simulink model "examples_of_product_block"  (R2021a)
settings: Solver=VariableStepAuto  StartTime=0.0  StopTime=1  RelTol=1e-3
settings Model: Creator=YasserNet  LastModifiedBy=YasserNet

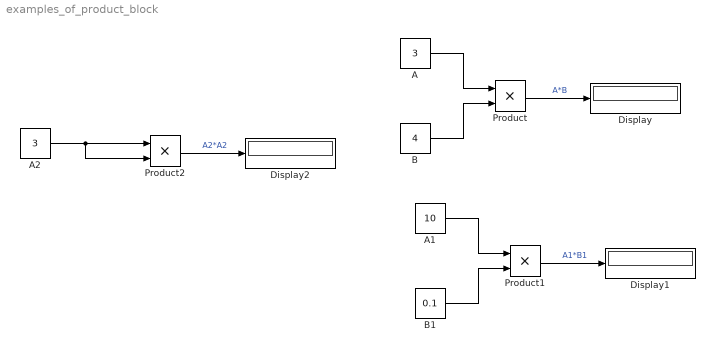
== system examples_of_product_block ==
  A : Constant  Value=3
  A1 : Constant  Value=10
  A2 : Constant  Value=3
  B : Constant  Value=4
  B1 : Constant  Value=0.1
  Display : Display
  Display1 : Display
  Display2 : Display
  Product : Product
  Product1 : Product
  Product2 : Product
  wires:
  Product/1 -> Display/1  "A*B"
  A/1 -> Product/1
  B/1 -> Product/2
  A1/1 -> Product1/1
  Product1/1 -> Display1/1  "A1*B1"
  B1/1 -> Product1/2
  A2/1 -> Product2/2, Product2/1
  Product2/1 -> Display2/1  "A2*A2"
